simulink model "BiCopter_Control_V1"  (R2022a)
settings: Solver=VariableStepAuto  StartTime=0.0  StopTime=10.0  RelTol=1e-3
values from neighbouring files (symbols this model uses):
  At = [0 1; 0 0]    [BiCopter_V0.m]    (also in BiCopter_runner.m)
  Bt = [0;1/J]    [BiCopter_V0.m]    (also in BiCopter_runner.m)
  C = [eye(2) zeros(2)]    [BiCopter_V0.m]    (also in BiCopter_runner.m)
  Ct = [1 0]    [BiCopter_V0.m]    (also in BiCopter_runner.m)
  Kq = Ka(:,5:6)    [BiCopter_V0.m]    (also in BiCopter_runner.m)
  Ktq = Kta(:,3)    [BiCopter_V0.m]    (also in BiCopter_runner.m)
  Ktx = Kta(:,1:2)    [BiCopter_V0.m]    (also in BiCopter_runner.m)
  Kx = Ka(:,1:4)    [BiCopter_V0.m]    (also in BiCopter_runner.m)
  m = 2    [BiCopter_V0.m]    (also in BiCopter_runner.m)
  theta_r = rand(1,1)    [BiCopter_V0.m]    (also in BiCopter_runner.m)
  x_r = rand(2,1)    [BiCopter_V0.m]    (also in BiCopter_runner.m = randn(2,1))
settings Model: Creator=Ankit  LastModifiedBy=Ankit

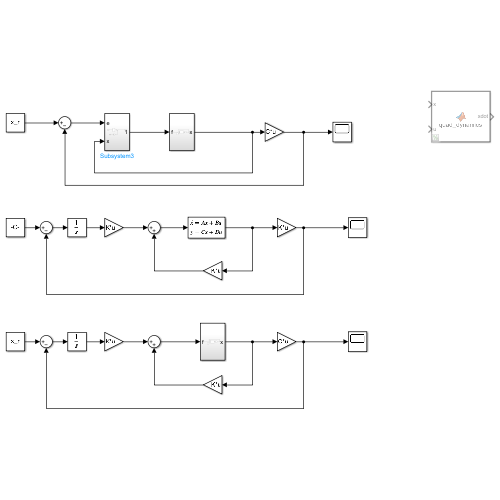
[thumbnail: Simulink's stored preview of the top-level diagram]
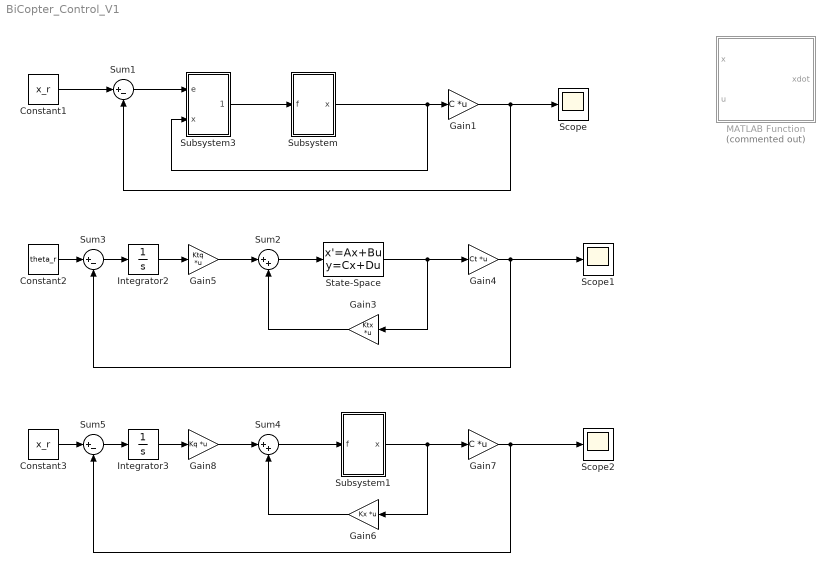
== system BiCopter_Control_V1 ==
  Constant1 : Constant  Value=x_r
  Constant2 : Constant  Value=theta_r
  Constant3 : Constant  Value=x_r
  Gain1 : Gain  Gain=C  Multiplication=Matrix(K*u)
  Gain3 : Gain  Gain=Ktx  Multiplication=Matrix(K*u)
  Gain4 : Gain  Gain=Ct  Multiplication=Matrix(K*u)
  Gain5 : Gain  Gain=Ktq  Multiplication=Matrix(K*u)
  Gain6 : Gain  Gain=Kx  Multiplication=Matrix(K*u)
  Gain7 : Gain  Gain=C  Multiplication=Matrix(K*u)
  Gain8 : Gain  Gain=Kq  Multiplication=Matrix(K*u)
  Integrator2 : Integrator
  Integrator3 : Integrator
  MATLAB Function : MATLAB Function  Commented=on  TreatAsAtomicUnit=on
  Scope : Scope
  Scope1 : Scope
  Scope2 : Scope
  State-Space : StateSpace  A=At  B=Bt  C=eye(2)  D=zeros(2,1)  InitialCondition=0
  Subsystem : Subsystem
  Subsystem1 : Subsystem
  Subsystem3 : Subsystem
  Sum1 : Sum  Inputs=|+-
  Sum2 : Sum  Inputs=|++
  Sum3 : Sum  Inputs=|+-
  Sum4 : Sum  Inputs=|++
  Sum5 : Sum  Inputs=|+-
  wires:
  Gain1/1 -> Scope/1, Sum1/2
  Constant1/1 -> Sum1/1
  Subsystem/1(x) -> Gain1/1, Subsystem3/2(x)
  Gain3/1 -> Sum2/2
  Gain4/1 -> Scope1/1, Sum3/2
  State-Space/1 -> Gain3/1, Gain4/1
  Gain5/1 -> Sum2/1
  Integrator2/1 -> Gain5/1
  Sum3/1 -> Integrator2/1
  Sum2/1 -> State-Space/1
  Constant2/1 -> Sum3/1
  Gain6/1 -> Sum4/2
  Gain7/1 -> Scope2/1, Sum5/2
  Subsystem1/1(x) -> Gain6/1, Gain7/1
  Gain8/1 -> Sum4/1
  Integrator3/1 -> Gain8/1
  Sum5/1 -> Integrator3/1
  Sum4/1 -> Subsystem1/1(f)
  Constant3/1 -> Sum5/1
  Sum1/1 -> Subsystem3/1(e)
  Subsystem3/1(Out1) -> Subsystem/1(f)

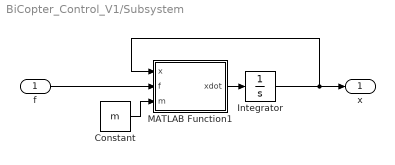
== system BiCopter_Control_V1/Subsystem ==
  f : Inport
  Constant : Constant  Value=m
  Integrator : Integrator
  MATLAB Function1 : MATLAB Function  TreatAsAtomicUnit=on
  x : Outport
  wires:
  Constant/1 -> MATLAB Function1/3(m)
  MATLAB Function1/1(xdot) -> Integrator/1
  f/1 -> MATLAB Function1/2(f)
  Integrator/1 -> MATLAB Function1/1(x), x/1

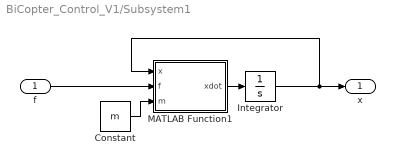
== system BiCopter_Control_V1/Subsystem1 ==
  f : Inport
  Constant : Constant  Value=m
  Integrator : Integrator
  MATLAB Function1 : MATLAB Function  TreatAsAtomicUnit=on
  x : Outport
  wires:
  Constant/1 -> MATLAB Function1/3(m)
  MATLAB Function1/1(xdot) -> Integrator/1
  f/1 -> MATLAB Function1/2(f)
  Integrator/1 -> MATLAB Function1/1(x), x/1

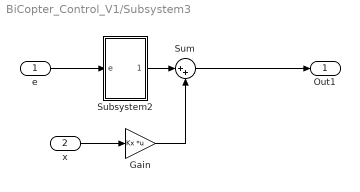
== system BiCopter_Control_V1/Subsystem3 ==
  e : Inport
  x : Inport  Port=2
  Gain : Gain  Gain=Kx  Multiplication=Matrix(K*u)
  Subsystem2 : Subsystem
  Sum : Sum  Inputs=|++
  Out1 : Outport
  wires:
  e/1 -> Subsystem2/1(e)
  Gain/1 -> Sum/2
  Subsystem2/1(u_int) -> Sum/1
  x/1 -> Gain/1
  Sum/1 -> Out1/1

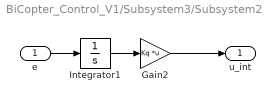
== system BiCopter_Control_V1/Subsystem3/Subsystem2 ==
  e : Inport
  Gain2 : Gain  Gain=Kq  Multiplication=Matrix(K*u)
  Integrator1 : Integrator
  u_int : Outport
  wires:
  Integrator1/1 -> Gain2/1
  Gain2/1 -> u_int/1
  e/1 -> Integrator1/1

== matlab function BiCopter_Control_V1/MATLAB Function ==
  data: x input; u input; xdot output
function xdot  = quad_dynamics(x,u)

m = 1;
J = blkdiag(10,10,1);

r = x(1:3,1);
v = x(4:6,1);

Eul_Angles = x(7:9,1);
omega_QE = x(10:12,1);

force = u(1);
moment = u(2:4);

g = [0;0;10];

xdot = x*0;

Phi     = Eul_Angles(1);
Theta   = Eul_Angles(2);
Psi     = Eul_Angles(3);


[O3psi, O2theta, O1phi] = orientation_matrices(Phi, Theta, Psi);

xdot(1:3,1) = v;
xdot(4:6,1) = g + force/m*transpose(O3psi) * transpose(O2theta) * transpose(O1phi)*[0;0;1];

xdot(7:9,1) = S_Phi_Theta_inv(Phi,Theta)*omega_QE;
xdot(10:12,1) = J\(-cross(omega_QE,J*omega_QE)+moment);


end

function S = S_Phi_Theta_inv(Phi,Theta)
S = [1 sin(Phi)*tan(Theta) cos(Phi)*tan(Theta);
    0 cos(Phi) -sin(Phi);
    0 sin(Phi)*sec(Theta) cos(Phi)*sec(Theta)];
end

function [O3psi, O2theta, O1phi] = orientation_matrices(phi, theta, psi);
O3psi = [cos(psi) sin(psi) 0;
    -sin(psi) cos(psi) 0;
    0 0 1];
O2theta = [cos(theta) 0 -sin(theta);
    0 1 0
    sin(theta) 0 cos(theta)];
O1phi = [1 0 0
    0 cos(phi) sin(phi);
    0 -sin(phi) cos(phi) ;];
end

== matlab function BiCopter_Control_V1/Subsystem1/MATLAB Function1 ==
  data: x input; xdot output; f input; m input
function xdot = fcn(x,f,m)

xdot = zeros(4,1);

xdot(1:2,1) = x(3:4,1);

xdot(3:4,1) = f/m+[0;10];

end

== matlab function BiCopter_Control_V1/Subsystem/MATLAB Function1 ==
  data: x input; xdot output; f input; m input
function xdot = fcn(x,f,m)

xdot = zeros(4,1);

xdot(1:2,1) = x(3:4,1);

xdot(3:4,1) = f/m+[0;10];

end
